simulink model "washing_machine"  (R2024b)
settings: Solver=VariableStepAuto  StartTime=0.0  StopTime=inf  RelTol=1e-3
settings Model: Creator=shiva  LastModifiedBy=shiva

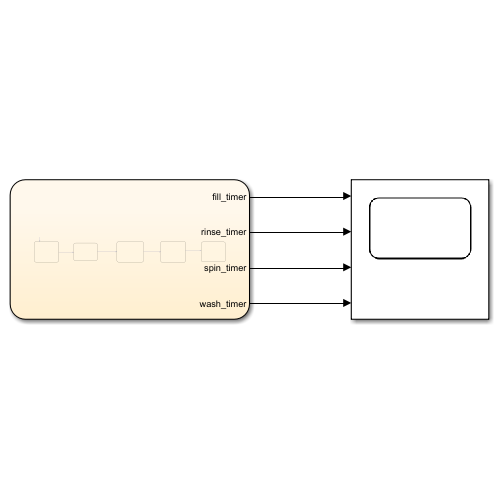
[thumbnail: Simulink's stored preview of the top-level diagram]
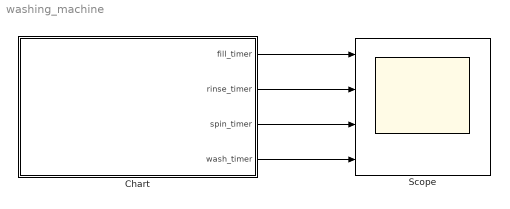
== system washing_machine ==
  Chart : Stateflow chart  TreatAsAtomicUnit=on
  Scope : Scope  NumInputPorts=4
  wires:
  Chart/1(fill_timer) -> Scope/1
  Chart/2(rinse_timer) -> Scope/2
  Chart/3(spin_timer) -> Scope/3
  Chart/4(wash_timer) -> Scope/4

== stateflow chart washing_machine/Chart ==
  state spin
    entry:
    spin_timer = 15;
    during:
    spin_timer = spin_timer - 1;
    exit:
    spin_timer = 0;
  state fill
    entry:
    fill_timer = 10;
    during:
    fill_timer = fill_timer - 1;
    exit:
    fill_timer = 0;
  state rinse
    entry:
    rinse_timer = 20;
    during:
    rinse_timer = rinse_timer - 1;
    exit:
    rinse_timer = 0;
  state done
    entry:
    disp('Cycle Complete');
  state wash
    entry:
    wash_timer = 30;
    during:
    wash_timer = wash_timer - 1;
    exit:
    wash_timer = 0;
  (default) -> fill
  spin -> done : [spin_timer<=0]
  wash -> rinse : [wash_timer<=0]
  rinse -> spin : [rinse_timer<=0]
  fill -> wash : [fill_timer <= 0]
  data: fill_timer output; rinse_timer output; spin_timer output; wash_timer output
